simulink model "control_block_diagram"  (R2025b)
settings: Solver=VariableStepAuto  StartTime=0.0  StopTime=10.0  RelTol=1e-3
InitFcn:
  | control_diagram_vars_and_functions
undefined symbols (not defined in the file): full_ROM, K_d, K_f, K_i, K_p, sine_freq_rad_s
settings Model: Creator=Madeline  LastModifiedBy=Madeline

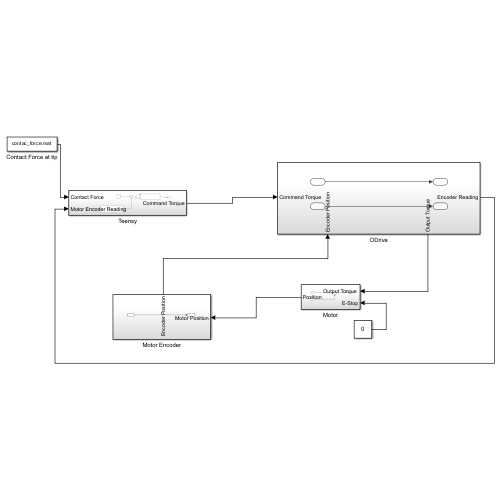
[thumbnail: Simulink's stored preview of the top-level diagram]
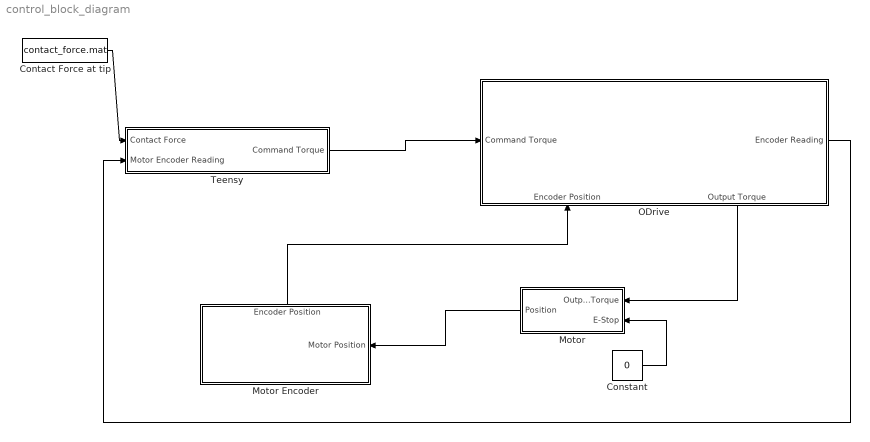
== system control_block_diagram ==
  Constant : Constant  Value=0
  Contact Force at tip : FromFile  FileName=contact_force.mat  SampleTime=0
  Motor : Subsystem
  Motor Encoder : Subsystem
      settings: PortSchema="{\"entries\":[{\"content\":{\"sides\":[{\"content\":{\"connectorIds\":[\"In1\"]},\"type\":\"ConnectorPlacement.EquallySpacedRectSide\",\"uuid\":\"88afd67f-3209-48d2-80be-27a9c6027e98\"},{\"content\":{\"side\":\"RIGHT\"},\"type\":\"ConnectorPlacement.EquallySpacedRectSide\",\"uuid\":\"6bd83a64-80e2-4e6b-a2e1-60e2a1b1e7d1\"},{\"content\":{\"connectorIds\":[\"Out1\"],\"side\":\"TOP\"},\"type\":\"ConnectorPlacement.EquallySpacedRectSide\",\"uuid\":\"ca5e5761-7c4c-4ffd-94f8-cf864c9b5854\"}]},\"type\":\"ConnectorPlacement.EquallySpacedConnector\",\"uuid\":\"578619f2-0797-4ece-88f8-3f0e3f24fe58\"}],\"packageUris\":[\"http://schema.mathworks.com/mf0/Connector/R2020b\"],\"version\":\"1.0\"}"
  ODrive : Subsystem
      settings: PortSchema="{\"entries\":[{\"content\":{\"sides\":[{\"content\":{\"connectorIds\":[\"In1\"]},\"type\":\"ConnectorPlacement.EquallySpacedRectSide\",\"uuid\":\"c97f3b25-cb08-4b77-804d-5691f1a52caa\"},{\"content\":{\"connectorIds\":[\"Out1\"],\"side\":\"RIGHT\"},\"type\":\"ConnectorPlacement.EquallySpacedRectSide\",\"uuid\":\"fc8ddf87-a458-4f73-a642-c7dd3d8cebff\"},{\"content\":{\"side\":\"TOP\"},\"type\":\"ConnectorPlacement.EquallySpacedRectSide\",\"uuid\":\"bec86457-f3cb-49fd-a085-c16f63c32d9e\"},{\"content\":{\"connectorIds\":[\"In2\",\"Out2\"],\"side\":\"BOTTOM\"},\"type\":\"ConnectorPlacement.EquallySpacedRectSide\",\"uuid\":\"4c0a5cbf-4f1d-4d43-a541-d1307432e3c9\"}]},\"type\":\"ConnectorPlacement.EquallySpacedConnector\",\"uuid\":\"94b3d347-19f8-405c-b5ff-c5a65504f3eb\"}],\"packageUris\":[\"http://schema.mathworks.com/mf0/Connector/R2020b\"],\"version\":\"1.0\"}"
  Teensy : Subsystem
  wires:
  ODrive/2("Output Torque ") -> Motor/1("Output Torque ")
  Motor/1("Position ") -> Motor Encoder/1(Motor Position)
  Teensy/1(Command Torque) -> ODrive/1(Command Torque)
  Contact Force at tip/1 -> Teensy/1(Contact Force)
  Motor Encoder/1(Encoder Position) -> ODrive/2(Encoder Position)
  ODrive/1(Encoder Reading) -> Teensy/2(Motor Encoder Reading)
  Constant/1 -> Motor/2(E-Stop)

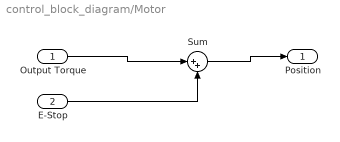
== system control_block_diagram/Motor ==
  "Output Torque " : Inport
  E-Stop : Inport  Port=2
  Sum : Sum  Inputs=|++
  "Position " : Outport
  wires:
  Sum/1 -> "Position "/1
  E-Stop/1 -> Sum/2
  "Output Torque "/1 -> Sum/1

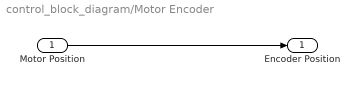
== system control_block_diagram/Motor Encoder ==
  Motor Position : Inport
  Encoder Position : Outport
  wires:
  Motor Position/1 -> Encoder Position/1

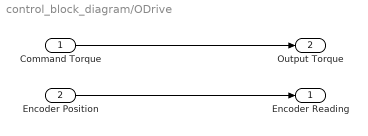
== system control_block_diagram/ODrive ==
  Command Torque : Inport
  Encoder Position : Inport  Port=2
  Encoder Reading : Outport
  "Output Torque " : Outport  Port=2
  wires:
  Command Torque/1 -> "Output Torque "/1
  Encoder Position/1 -> Encoder Reading/1

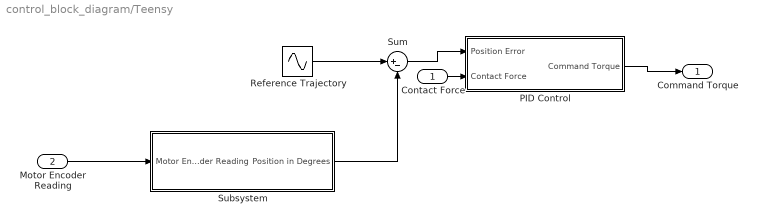
== system control_block_diagram/Teensy ==
  Contact Force : Inport
  Motor Encoder Reading : Inport  Port=2
  PID Control : Subsystem
  Reference Trajectory : Sin  Amplitude=0.75*full_ROM  Frequency=sine_freq_rad_s  SampleTime=0
  Subsystem : Subsystem
  Sum : Sum  Inputs=|+-
  Command Torque : Outport
  wires:
  Sum/1 -> PID Control/1(Position Error)
  PID Control/1(Command Torque) -> Command Torque/1
  Motor Encoder Reading/1 -> Subsystem/1(Motor Encoder Reading)
  Reference Trajectory/1 -> Sum/1
  Contact Force/1 -> PID Control/2(Contact Force)
  Subsystem/1(Position in Degrees) -> Sum/2

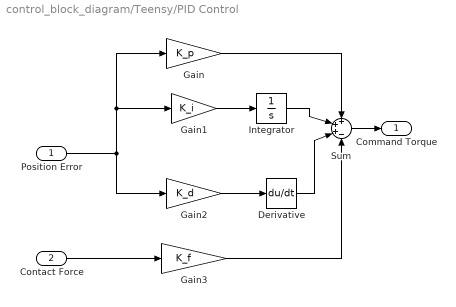
== system control_block_diagram/Teensy/PID Control ==
  Position Error : Inport
  Contact Force : Inport  Port=2
  Derivative : Derivative
  Gain : Gain  Gain=K_p
  Gain1 : Gain  Gain=K_i
  Gain2 : Gain  Gain=K_d
  Gain3 : Gain  Gain=K_f
  Integrator : Integrator
  Sum : Sum  Inputs=+++-
  Command Torque : Outport
  wires:
  Position Error/1 -> Gain2/1, Gain/1, Gain1/1
  Gain2/1 -> Derivative/1
  Gain1/1 -> Integrator/1
  Gain/1 -> Sum/1
  Integrator/1 -> Sum/2
  Derivative/1 -> Sum/3
  Sum/1 -> Command Torque/1
  Contact Force/1 -> Gain3/1
  Gain3/1 -> Sum/4

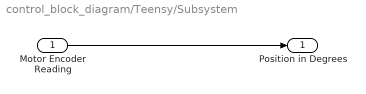
== system control_block_diagram/Teensy/Subsystem ==
  Motor Encoder Reading : Inport
  Position in Degrees : Outport
  wires:
  Motor Encoder Reading/1 -> Position in Degrees/1
